simulink library "INP_BRK_Prep"  (R2024b)
settings: Solver=VariableStepAuto  StartTime=0.0  StopTime=10.0  RelTol=1e-3
undefined symbols (not defined in the file): INP_BRK_p_PresBrkFrOfs_bar, INP_BRK_p_PresBrkFrSca_na, INP_BRK_p_PresBrkReOfs_bar, INP_BRK_p_PresBrkReSca_na, INP_c_TiSample_s, INP_p_TiTau_s
libraries: VUT_lib x2
settings Model: Creator=blatak  LastModifiedBy=blatak

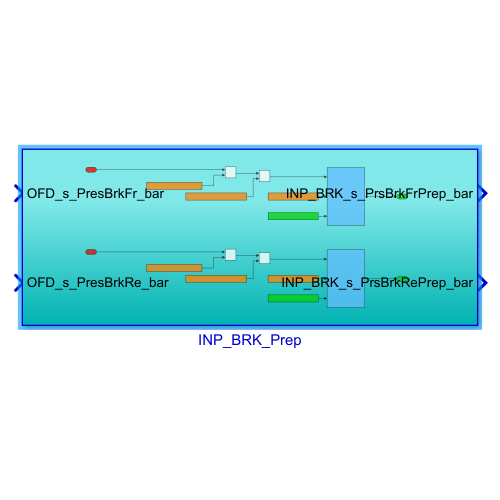
[thumbnail: Simulink's stored preview of the top-level diagram]
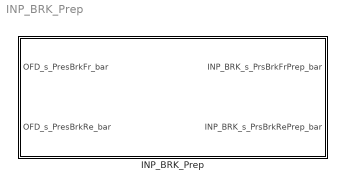
== system INP_BRK_Prep ==
  INP_BRK_Prep : Subsystem

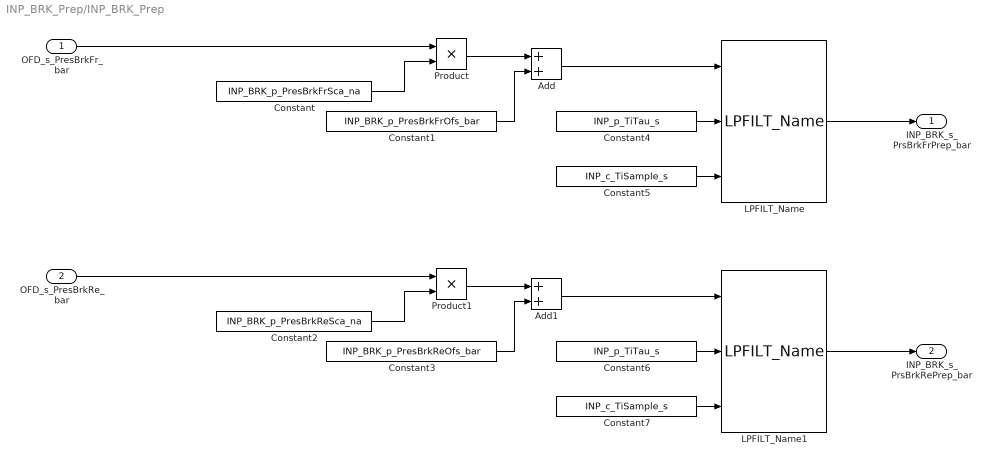
== system INP_BRK_Prep/INP_BRK_Prep ==
  OFD_s_PresBrkFr_bar : Inport  Description=Front brake pressure - raw measured value
  OFD_s_PresBrkRe_bar : Inport  Description=Front brake pressure - raw measured value  Port=2
  Add : Sum
  Add1 : Sum
  Constant : Constant  Description=Scaling coefficient to recalculate the electric quantity to the physical one - longitudinal acceleration  Value=INP_BRK_p_PresBrkFrSca_na
  Constant1 : Constant  Description=Offset to recalculate the electric quantity to the physical one - longitudinal acceleration  Value=INP_BRK_p_PresBrkFrOfs_bar
  Constant2 : Constant  Description=Scaling coefficient to recalculate the electric quantity to the physical one - longitudinal acceleration  Value=INP_BRK_p_PresBrkReSca_na
  Constant3 : Constant  Description=Offset to recalculate the electric quantity to the physical one - longitudinal acceleration  Value=INP_BRK_p_PresBrkReOfs_bar
  Constant4 : Constant  Value=INP_p_TiTau_s
  Constant5 : Constant  Value=INP_c_TiSample_s
  Constant6 : Constant  Value=INP_p_TiTau_s
  Constant7 : Constant  Value=INP_c_TiSample_s
  LPFILT_Name : VUT_lib/LPFILT_Name  SystemSampleTime=-1  VariantActivationTime=update diagram  AllowFlexibleInterface=on  Latency=0  AutoFrameSizeCalculation=off
  LPFILT_Name1 : VUT_lib/LPFILT_Name  SystemSampleTime=-1  VariantActivationTime=update diagram  AllowFlexibleInterface=on  Latency=0  AutoFrameSizeCalculation=off
  Product : Product
  Product1 : Product
  INP_BRK_s_PrsBrkFrPrep_bar : Outport  Description=INP Front brake pressure - value after basic processing, filtering, scale, offset - if necessary
  INP_BRK_s_PrsBrkRePrep_bar : Outport  Description=INP Front brake pressure - value after basic processing, filtering, scale, offset - if necessary  Port=2
  wires:
  Constant/1 -> Product/2
  OFD_s_PresBrkRe_bar/1 -> Product1/1
  OFD_s_PresBrkFr_bar/1 -> Product/1
  Product1/1 -> Add1/1
  Add1/1 -> LPFILT_Name1/1
  Constant3/1 -> Add1/2
  LPFILT_Name1/1 -> INP_BRK_s_PrsBrkRePrep_bar/1
  Constant6/1 -> LPFILT_Name1/2
  Constant7/1 -> LPFILT_Name1/3
  Constant2/1 -> Product1/2
  Constant4/1 -> LPFILT_Name/2
  Add/1 -> LPFILT_Name/1
  Constant5/1 -> LPFILT_Name/3
  Product/1 -> Add/1
  LPFILT_Name/1 -> INP_BRK_s_PrsBrkFrPrep_bar/1
  Constant1/1 -> Add/2
